simulink model "Test_Wiper_Model"  (R2024a)
settings: Solver=VariableStepAuto  StartTime=0.0  StopTime=10.0  RelTol=1e-3
settings Model: Creator=ec97883  LastModifiedBy=ec97883

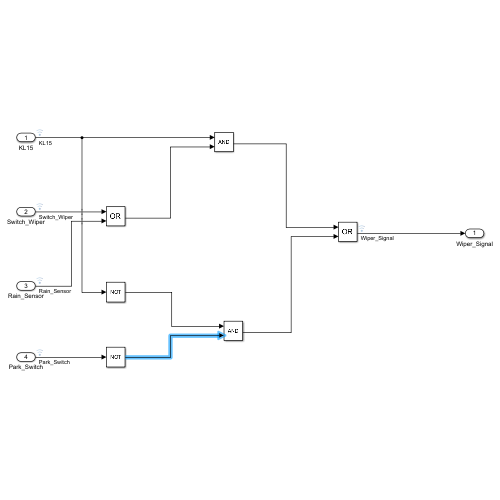
[thumbnail: Simulink's stored preview of the top-level diagram]
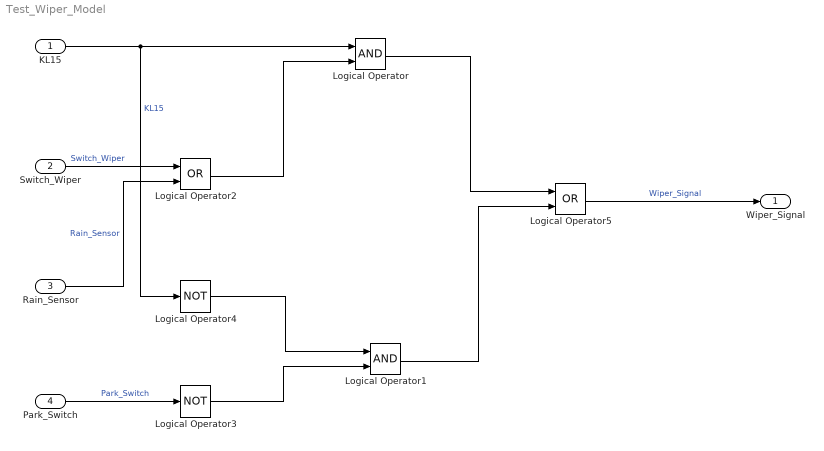
== system Test_Wiper_Model ==
  KL15 : Inport  OutDataTypeStr=boolean  PortDimensions=1
  Switch_Wiper : Inport  Port=2  OutDataTypeStr=boolean  PortDimensions=1
  Rain_Sensor : Inport  Port=3  OutDataTypeStr=boolean  PortDimensions=1
  Park_Switch : Inport  Port=4  OutDataTypeStr=boolean  PortDimensions=1
  Logical Operator : Logic  AllPortsSameDT=off  OutDataTypeStr=boolean
  Logical Operator1 : Logic  AllPortsSameDT=off  OutDataTypeStr=boolean
  Logical Operator2 : Logic  Operator=OR  AllPortsSameDT=off  OutDataTypeStr=boolean
  Logical Operator3 : Logic  Operator=NOT  AllPortsSameDT=off  OutDataTypeStr=boolean
  Logical Operator4 : Logic  Operator=NOT  AllPortsSameDT=off  OutDataTypeStr=boolean
  Logical Operator5 : Logic  Operator=OR  AllPortsSameDT=off  OutDataTypeStr=boolean
  Wiper_Signal : Outport  OutDataTypeStr=boolean  PortDimensions=1
  wires:
  KL15/1 -> Logical Operator4/1, Logical Operator/1  "KL15"
  Switch_Wiper/1 -> Logical Operator2/1  "Switch_Wiper"
  Logical Operator2/1 -> Logical Operator/2
  Rain_Sensor/1 -> Logical Operator2/2  "Rain_Sensor"
  Park_Switch/1 -> Logical Operator3/1  "Park_Switch"
  Logical Operator4/1 -> Logical Operator1/1
  Logical Operator/1 -> Logical Operator5/1
  Logical Operator1/1 -> Logical Operator5/2
  Logical Operator5/1 -> Wiper_Signal/1  "Wiper_Signal"
  Logical Operator3/1 -> Logical Operator1/2
